simulink model "AlexFullVehicleModel2018"  (R2018b)
settings: Solver=FixedStepAuto  StartTime=0.0  StopTime=20  FixedStep=global_time_step  MaxStep=0.05  RelTol=1e-3
values from neighbouring files (symbols this model uses):
  B_lat = @(i,u,v)feval(B_surf_lat{i},[u,v])    [initfunctions.m]
  B_long = @(i,u,v)feval(B_surf_long{i},[u,v])    [initfunctions.m]
  brake_bias = 0.6    [fvm_parameters.m]
  brake_pad_radius = 0.1    [fvm_parameters.m]
  C_lat = @(i,u,v)feval(C_surf_lat{i},[u,v])    [initfunctions.m]
  C_long = @(i,u,v)feval(C_surf_long{i},[u,v])    [initfunctions.m]
  D_lat = @(i,u,v)feval(D_surf_lat{i},[u,v])    [initfunctions.m]
  D_long = @(i,u,v)feval(D_surf_long{i},[u,v])    [initfunctions.m]
  E_lat = @(i,u,v)feval(E_surf_lat{i},[u,v])    [initfunctions.m]
  E_long = @(i,u,v)feval(E_surf_long{i},[u,v])    [initfunctions.m]
  front_piston_area = 1.555284713E-3    (= 0.001555284713)    [fvm_parameters.m]
  master_cylinder_area = 3.3329E-4    (= 0.00033329)    [fvm_parameters.m]
  mu_brake = 0.35    [fvm_parameters.m]
  Mu_lat = @(i,u,v)feval(Mu_surf_lat{i},[u,v])    [initfunctions.m]
  Mu_long = @(i,u,v)feval(Mu_surf_long{i},[u,v])    [initfunctions.m]
  n_pads = 2    [fvm_parameters.m]
  pedal_ratio = 5.22    [fvm_parameters.m]
  rear_piston_area = 1.017876020E-3    (= 0.00101787602)    [fvm_parameters.m]
undefined symbols (not defined in the file or in its folder): sigbuilder_block
libraries: cstblocks x1
settings Model: Creator=jbray  LastModifiedBy=univ4123
settings SolverCC: InitialStep=0.001
settings DataIOCC: ReturnWorkspaceOutputs=on
settings DebuggingCC: UnderSpecifiedDimensionMsg=warning

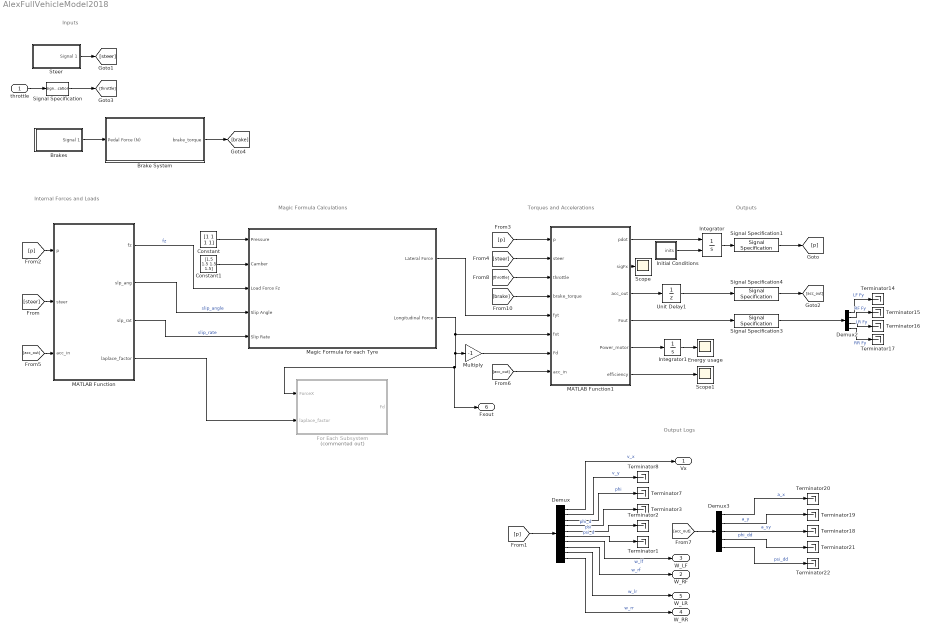
== system AlexFullVehicleModel2018 ==
  note: Torques and Accelerations
  note: Internal Forces and Loads
  note: Outputs
  note: Output Logs
  note: Magic Formula Calculations
  note: Inputs
  throttle : Inport
  Brake System : Subsystem
  Brakes : Subsystem  Tag=STV Subsys  LoadFcn=sigbuilder_block('load');  StartFcn=sigbuilder_block('start');  StopFcn=sigbuilder_block('stop');  ClipboardFcn=sigbuilder_block('clipboard');  mask(Sigbuilder block){tuvar=[0:10]}
      mask help: Simulink:masks:SigbuilderBlock_MD
      mask init:
      | if ~strcmp(get_param(bdroot(gcbh),'SimulationStatus'),'stopped') tuvar = sigbuilder_block('maskInit'); end
      settings: CopyFcn=sigbuilder_block('copy');  DeleteFcn=sigbuilder_block('delete');  ModelCloseFcn=sigbuilder_block('modelClose');  PreSaveFcn=sigbuilder_block('preSave');  PauseFcn=sigbuilder_block('pause');  ContinueFcn=sigbuilder_block('continue');  NameChangeFcn=sigbuilder_block('namechange');  OpenFcn=sigbuilder_block('open',[404 117.5 550.5 362.5 ]);  CloseFcn=sigbuilder_block('close');
      mask Display: plot(0, 0, 100, 100,[2, 2, 32, 32, 2], [68, 8, 8, 68, 68],[32, 2], [38, 38], [32, 19, 2],[53, 60, 44], [32, 17, 17, 2],[16, 16, 31, 31]);txt = getActiveGroup(gcbh);text(2, 100, txt,'verticalAlignment', 'top');
  Constant : Constant  Value=[1 1 1 1]  VectorParams1D=off  LockScale=on
  Constant1 : Constant  Value=[1.5 1.5 1.5 1.5]  VectorParams1D=off  LockScale=on
  Demux : Demux  Outputs=10
  Demux2 : Demux
  Demux3 : Demux  Outputs=5
  Energy usage : Scope
  For Each Subsystem : Subsystem  Commented=on  TreatAsAtomicUnit=on
  "Initial Conditions " : Subsystem
  Integrator : Integrator  InitialConditionSource=external
  Integrator1 : Integrator
  MATLAB Function : MATLAB Function  TreatAsAtomicUnit=on
  MATLAB Function1 : MATLAB Function  TreatAsAtomicUnit=on
  Magic Formula for each Tyre : Subsystem  TreatAsAtomicUnit=on
  Multiply : Gain  Gain=-1
  Scope : Scope
  Scope1 : Scope
  Signal Specification : SignalSpecification  Dimensions=[2,1]
  Signal Specification1 : SignalSpecification  Dimensions=10
  Signal Specification3 : SignalSpecification  Dimensions=4
  Signal Specification4 : SignalSpecification  Dimensions=5
  "Steer " : Subsystem  Tag=STV Subsys  LoadFcn=sigbuilder_block('load');  StartFcn=sigbuilder_block('start');  StopFcn=sigbuilder_block('stop');  ClipboardFcn=sigbuilder_block('clipboard');  mask(Sigbuilder block){tuvar=[0:10]}
      mask help: Simulink:masks:SigbuilderBlock_MD
      mask init:
      | if ~strcmp(get_param(bdroot(gcbh),'SimulationStatus'),'stopped') tuvar = sigbuilder_block('maskInit'); end
      settings: CopyFcn=sigbuilder_block('copy');  DeleteFcn=sigbuilder_block('delete');  ModelCloseFcn=sigbuilder_block('modelClose');  PreSaveFcn=sigbuilder_block('preSave');  PauseFcn=sigbuilder_block('pause');  ContinueFcn=sigbuilder_block('continue');  NameChangeFcn=sigbuilder_block('namechange');  OpenFcn=sigbuilder_block('open',[404 117.5 550.5 362.5 ]);  CloseFcn=sigbuilder_block('close');
      mask Display: plot(0, 0, 100, 100,[2, 2, 32, 32, 2], [68, 8, 8, 68, 68],[32, 2], [38, 38], [32, 19, 2],[53, 60, 44], [32, 17, 17, 2],[16, 16, 31, 31]);txt = getActiveGroup(gcbh);text(2, 100, txt,'verticalAlignment', 'top');
  Terminator{1..3,7..8,14..22} (14 alike) : Terminator
  Unit Delay1 : UnitDelay  SampleTime=-1
  Vx : Outport
  W_RF : Outport  Port=2
  W_LF : Outport  Port=3
  W_RR : Outport  Port=4
  W_LR : Outport  Port=5
  Fxout : Outport  Port=6
  wires:
  MATLAB Function1/1(pdot) -> Integrator/1
  Integrator/1 -> Signal Specification1/1
  Demux/10 -> W_RR/1  "w_rr"
  Demux/9 -> W_LR/1  "w_lr"
  Demux/6 -> Terminator1/1  "psi_d"
  Demux/5 -> Terminator2/1  "psi"
  Demux/4 -> Terminator3/1  "phi_d"
  Demux/7 -> W_LF/1  "w_lf"
  Demux/8 -> W_RF/1  "w_rf"
  Demux/3 -> Terminator7/1  "phi"
  Demux/2 -> Terminator8/1  "v_y"
  Demux/1 -> Vx/1  "v_x"
  Demux2/4 -> Terminator17/1  "RR Fy"
  Demux2/3 -> Terminator16/1  "LR Fy"
  Demux2/2 -> Terminator15/1  "RF Fy"
  Demux2/1 -> Terminator14/1  "LF Fy"
  Signal Specification3/1 -> Demux2/1
  Demux3/3 -> Terminator18/1  "a_sy"
  Demux3/2 -> Terminator19/1  "a_y"
  Demux3/1 -> Terminator20/1  "a_x"
  Demux3/4 -> Terminator21/1  "phi_dd"
  Demux3/5 -> Terminator22/1  "psi_dd"
  MATLAB Function/3(slp_rat) -> Magic Formula for each Tyre/5(Slip Rate)  "slip_rate"
  MATLAB Function/1(fz) -> Magic Formula for each Tyre/3(Load Force Fz)  "fz"
  Constant/1 -> Magic Formula for each Tyre/1(Pressure)
  Magic Formula for each Tyre/1(Lateral Force) -> MATLAB Function1/5(fyt)
  Magic Formula for each Tyre/2(Longitudinal Force) -> MATLAB Function1/6(fxt), Multiply/1, Fxout/1, For Each Subsystem/1(ForceX)
  MATLAB Function1/3(acc_out) -> Unit Delay1/1
  MATLAB Function/2(slp_ang) -> Magic Formula for each Tyre/4(Slip Angle)  "slip_angle"
  Constant1/1 -> Magic Formula for each Tyre/2(Camber)
  MATLAB Function1/2(sigFx) -> Scope/1
  MATLAB Function/4(laplace_factor) -> For Each Subsystem/2(laplace_factor)
  Signal Specification1/1 -> [p]
  [p] -> Demux/1
  [p] -> MATLAB Function/1(p)
  [p] -> MATLAB Function1/1(p)
  [steer] -> MATLAB Function/2(steer)
  [steer] -> MATLAB Function1/2(steer)
  Unit Delay1/1 -> Signal Specification4/1
  Signal Specification4/1 -> [acc_out]
  [acc_out] -> MATLAB Function/3(acc_in)
  [acc_out] -> MATLAB Function1/8(acc_in)
  [acc_out] -> Demux3/1
  "Initial Conditions "/1("inits ") -> Integrator/2
  Multiply/1 -> MATLAB Function1/7(Fd)
  [throttle] -> MATLAB Function1/3(throttle)
  MATLAB Function1/5(Power_motor) -> Integrator1/1
  Integrator1/1 -> Energy usage/1
  MATLAB Function1/6(efficiency) -> Scope1/1
  "Steer "/1(Signal 1) -> [steer]
  throttle/1 -> Signal Specification/1
  Brakes/1(Signal 1) -> Brake System/1(Pedal Force (N))
  Brake System/1("brake_torque ") -> [brake]
  [brake] -> MATLAB Function1/4(brake_torque)
  MATLAB Function1/4(Fout) -> Signal Specification3/1
  Signal Specification/1 -> [throttle]

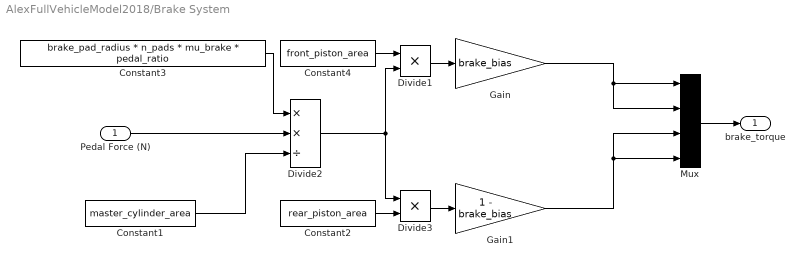
== system AlexFullVehicleModel2018/Brake System ==
  Pedal Force (N) : Inport
  Constant1 : Constant  Value=master_cylinder_area
  Constant2 : Constant  Value=rear_piston_area
  Constant3 : Constant  Value=brake_pad_radius * n_pads * mu_brake * pedal_ratio
  Constant4 : Constant  Value=front_piston_area
  Divide1 : Product
  Divide2 : Product  Inputs=**/
  Divide3 : Product
  Gain : Gain  Gain=brake_bias
  Gain1 : Gain  Gain=1 - brake_bias
  Mux : Mux
  "brake_torque " : Outport
  wires:
  Mux/1 -> "brake_torque "/1
  Divide1/1 -> Gain/1
  Pedal Force (N)/1 -> Divide2/2
  Constant1/1 -> Divide2/3
  Constant2/1 -> Divide3/2
  Divide2/1 -> Divide1/2, Divide3/1
  Divide3/1 -> Gain1/1
  Constant3/1 -> Divide2/1
  Gain/1 -> Mux/2, Mux/1
  Constant4/1 -> Divide1/1
  Gain1/1 -> Mux/4, Mux/3

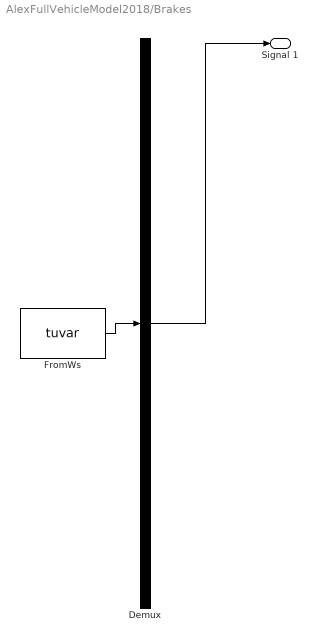
== system AlexFullVehicleModel2018/Brakes ==
  Demux : Demux  Tag=STV Demux  Outputs=1
  FromWs : FromWorkspace  Tag=STV FromWs  VariableName=tuvar  SampleTime=0
      SigBuilderData=|
      | common.afterFinalStr = 'Extrapolate'
      | common.sampleTime = 0
      | dataSet.timeRange = [0 20]
      | dataSet.name = 'Group 1'
      | sbobj.Groups.Name = 'Group 1'
      | sbobj.Groups.Signals.Name = 'Signal 1'
      | sbobj.Groups.Signals.XData = [0 9.02 14 17.25 20]
      | sbobj.Groups.Signals.YData = [0 0 0 0 0]
      | sbobj.Groups.TimeRange = [0 20]
  Signal 1 : Outport  Tag=STV Outport
  wires:
  Demux/1 -> Signal 1/1
  FromWs/1 -> Demux/1

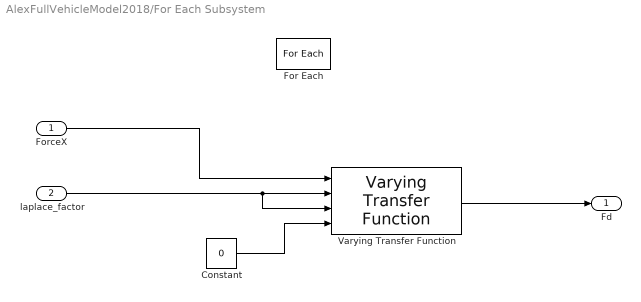
== system AlexFullVehicleModel2018/For Each Subsystem ==
  ForceX : Inport  Partition=on  PartitionDimension=1  PartitionWidth=1  PartitionOffset=0
  laplace_factor : Inport  Port=2  Partition=on  PartitionDimension=2  PartitionWidth=1  PartitionOffset=0
  Constant : Constant  Value=0
  For Each : ForEach  DisableCoverage=on  IndexMode=One-based
  Varying Transfer Function : cstblocks/Linear Parameter Varying/Varying Transfer Function  N=1
      settings: SourceProductName=Control System Toolbox
  "Fd " : Outport  ConcatenationDimension=1
  wires:
  Constant/1 -> Varying Transfer Function/4
  laplace_factor/1 -> Varying Transfer Function/3, Varying Transfer Function/2
  ForceX/1 -> Varying Transfer Function/1
  Varying Transfer Function/1 -> "Fd "/1

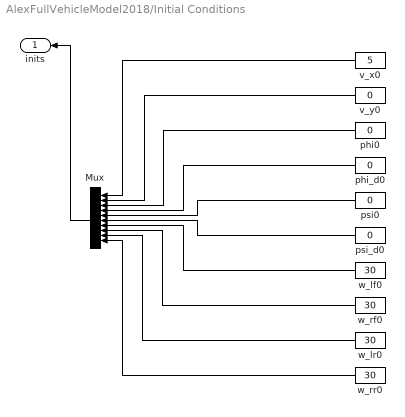
== system AlexFullVehicleModel2018/Initial Conditions  ==
  Mux : Mux  Inputs=10
  phi0 : Constant  Value=0
  phi_d0 : Constant  Value=0
  psi0 : Constant  Value=0
  psi_d0 : Constant  Value=0
  v_x0 : Constant  Value=5
  v_y0 : Constant  Value=0
  w_lf0 : Constant  Value=30
  w_lr0 : Constant  Value=30
  w_rf0 : Constant  Value=30
  w_rr0 : Constant  Value=30
  "inits " : Outport
  wires:
  w_lf0/1 -> Mux/7
  Mux/1 -> "inits "/1
  psi_d0/1 -> Mux/6
  psi0/1 -> Mux/5
  phi_d0/1 -> Mux/4
  phi0/1 -> Mux/3
  v_y0/1 -> Mux/2
  w_rf0/1 -> Mux/8
  v_x0/1 -> Mux/1
  w_rr0/1 -> Mux/10
  w_lr0/1 -> Mux/9

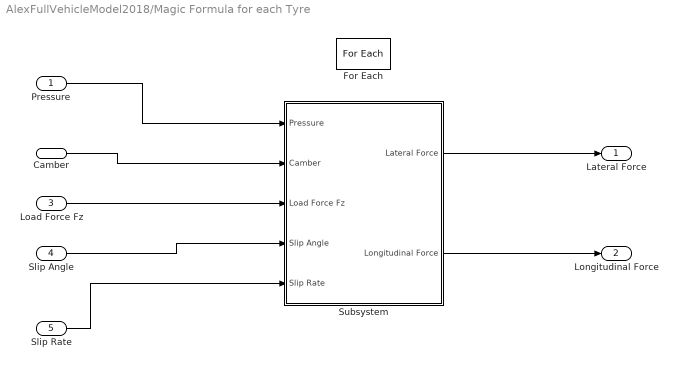
== system AlexFullVehicleModel2018/Magic Formula for each Tyre ==
  Pressure : Inport  Partition=on  PartitionDimension=2  PartitionWidth=1  PartitionOffset=0
  Camber : Inport  Port=2  Partition=on  PartitionDimension=2  PartitionWidth=1  PartitionOffset=0
  Load Force Fz : Inport  Port=3  Partition=on  PartitionDimension=2  PartitionWidth=1  PartitionOffset=0
  Slip Angle : Inport  Port=4  Partition=on  PartitionDimension=2  PartitionWidth=1  PartitionOffset=0
  Slip Rate : Inport  Port=5  Partition=on  PartitionDimension=2  PartitionWidth=1  PartitionOffset=0
  For Each : ForEach  DisableCoverage=on  IndexMode=One-based
  Subsystem : Subsystem
  Lateral Force : Outport  ConcatenationDimension=1
  Longitudinal Force : Outport  Port=2  ConcatenationDimension=1
  wires:
  Slip Rate/1 -> Subsystem/5(Slip Rate)
  Slip Angle/1 -> Subsystem/4(Slip Angle)
  Pressure/1 -> Subsystem/1(Pressure)
  Subsystem/1(Lateral Force) -> Lateral Force/1
  Load Force Fz/1 -> Subsystem/3(Load Force Fz)
  Camber/1 -> Subsystem/2(Camber)
  Subsystem/2(Longitudinal Force) -> Longitudinal Force/1

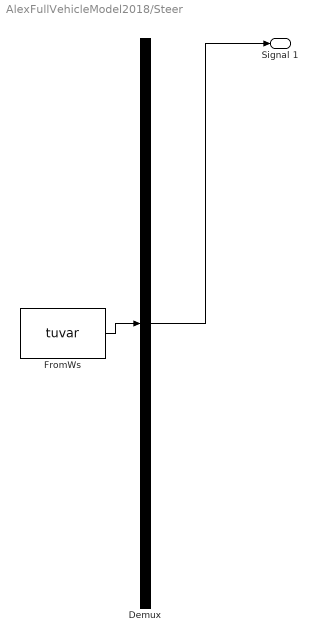
== system AlexFullVehicleModel2018/Steer  ==
  Demux : Demux  Tag=STV Demux  Outputs=1
  FromWs : FromWorkspace  Tag=STV FromWs  VariableName=tuvar  SampleTime=0
      SigBuilderData=|
      | common.afterFinalStr = 'Extrapolate'
      | common.sampleTime = 0
      | dataSet.timeRange = [0 20]
      | dataSet.name = 'Group 1'
      | sbobj.Groups.Name = 'Group 1'
      | sbobj.Groups.Signals.Name = 'Signal 1'
      | sbobj.Groups.Signals.XData = [0 4 6 16 20]
      | sbobj.Groups.Signals.YData = [0 0 0 0 0]
      | sbobj.Groups.TimeRange = [0 20]
  Signal 1 : Outport  Tag=STV Outport
  wires:
  Demux/1 -> Signal 1/1
  FromWs/1 -> Demux/1

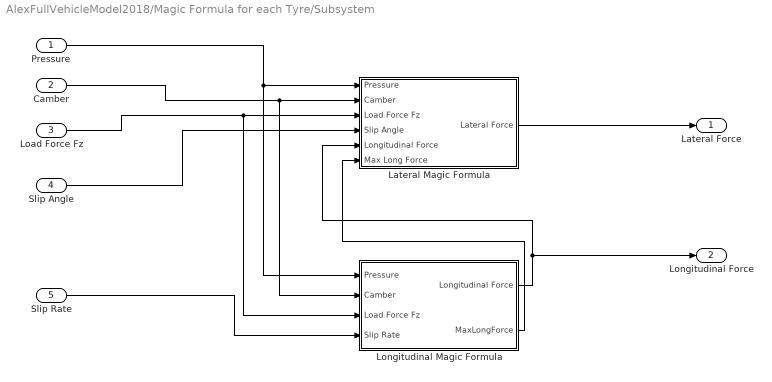
== system AlexFullVehicleModel2018/Magic Formula for each Tyre/Subsystem ==
  Pressure : Inport
  Camber : Inport  Port=2
  Load Force Fz : Inport  Port=3
  Slip Angle : Inport  Port=4
  Slip Rate : Inport  Port=5
  Lateral Magic Formula : Subsystem
  Longitudinal Magic Formula : Subsystem
  Lateral Force : Outport
  Longitudinal Force : Outport  Port=2
  wires:
  Slip Angle/1 -> Lateral Magic Formula/4(Slip Angle)
  Lateral Magic Formula/1(Lateral Force) -> Lateral Force/1
  Load Force Fz/1 -> Longitudinal Magic Formula/3(Load Force Fz), Lateral Magic Formula/3(Load Force Fz)
  Longitudinal Magic Formula/1(Longitudinal Force) -> Lateral Magic Formula/5(Longitudinal Force), Longitudinal Force/1
  Camber/1 -> Longitudinal Magic Formula/2(Camber), Lateral Magic Formula/2(Camber)
  Slip Rate/1 -> Longitudinal Magic Formula/4(Slip Rate)
  Pressure/1 -> Longitudinal Magic Formula/1(Pressure), Lateral Magic Formula/1(Pressure)
  Longitudinal Magic Formula/2("MaxLongForce ") -> Lateral Magic Formula/6(Max Long Force)

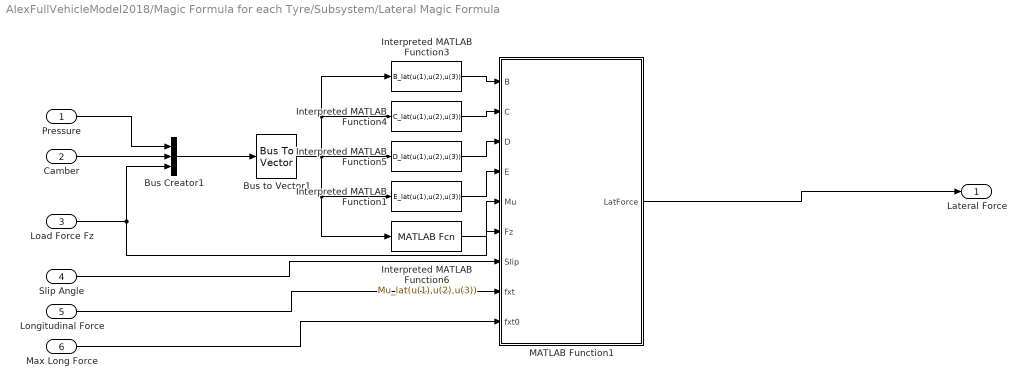
== system AlexFullVehicleModel2018/Magic Formula for each Tyre/Subsystem/Lateral Magic Formula ==
  Pressure : Inport
  Camber : Inport  Port=2
  Load Force Fz : Inport  Port=3
  Slip Angle : Inport  Port=4
  Longitudinal Force : Inport  Port=5
  Max Long Force : Inport  Port=6
  Bus Creator1 : BusCreator  Inputs=3
  Bus to Vector1 : BusToVector
  Interpreted MATLAB Function1 : MATLABFcn  MATLABFcn=E_lat(u(1),u(2),u(3))
  Interpreted MATLAB Function3 : MATLABFcn  MATLABFcn=B_lat(u(1),u(2),u(3))
  Interpreted MATLAB Function4 : MATLABFcn  MATLABFcn=C_lat(u(1),u(2),u(3))
  Interpreted MATLAB Function5 : MATLABFcn  MATLABFcn=D_lat(u(1),u(2),u(3))
  Interpreted MATLAB Function6 : MATLABFcn  MATLABFcn=Mu_lat(u(1),u(2),u(3))
  MATLAB Function1 : MATLAB Function  TreatAsAtomicUnit=on
  Lateral Force : Outport
  wires:
  Interpreted MATLAB Function3/1 -> MATLAB Function1/1(B)
  Interpreted MATLAB Function1/1 -> MATLAB Function1/4(E)
  Bus to Vector1/1 -> Interpreted MATLAB Function1/1, Interpreted MATLAB Function6/1, Interpreted MATLAB Function3/1, Interpreted MATLAB Function4/1, Interpreted MATLAB Function5/1
  Load Force Fz/1 -> Bus Creator1/3, MATLAB Function1/6(Fz)
  Interpreted MATLAB Function4/1 -> MATLAB Function1/2(C)
  Slip Angle/1 -> MATLAB Function1/7(Slip)
  Interpreted MATLAB Function5/1 -> MATLAB Function1/3(D)
  Pressure/1 -> Bus Creator1/1
  Interpreted MATLAB Function6/1 -> MATLAB Function1/5(Mu)
  Bus Creator1/1 -> Bus to Vector1/1
  Camber/1 -> Bus Creator1/2
  MATLAB Function1/1(LatForce) -> Lateral Force/1
  Longitudinal Force/1 -> MATLAB Function1/8(fxt)
  Max Long Force/1 -> MATLAB Function1/9(fxt0)

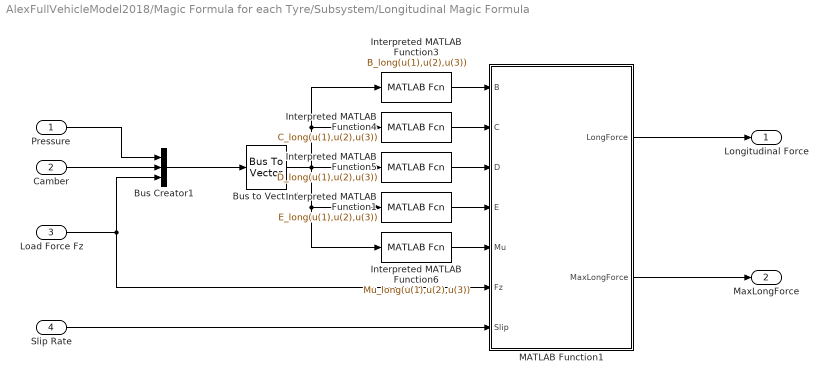
== system AlexFullVehicleModel2018/Magic Formula for each Tyre/Subsystem/Longitudinal Magic Formula ==
  Pressure : Inport
  Camber : Inport  Port=2
  Load Force Fz : Inport  Port=3
  Slip Rate : Inport  Port=4
  Bus Creator1 : BusCreator  Inputs=3
  Bus to Vector1 : BusToVector
  Interpreted MATLAB Function1 : MATLABFcn  MATLABFcn=E_long(u(1),u(2),u(3))
  Interpreted MATLAB Function3 : MATLABFcn  MATLABFcn=B_long(u(1),u(2),u(3))
  Interpreted MATLAB Function4 : MATLABFcn  MATLABFcn=C_long(u(1),u(2),u(3))
  Interpreted MATLAB Function5 : MATLABFcn  MATLABFcn=D_long(u(1),u(2),u(3))
  Interpreted MATLAB Function6 : MATLABFcn  MATLABFcn=Mu_long(u(1),u(2),u(3))
  MATLAB Function1 : MATLAB Function  TreatAsAtomicUnit=on
  Longitudinal Force : Outport
  "MaxLongForce " : Outport  Port=2
  wires:
  Interpreted MATLAB Function3/1 -> MATLAB Function1/1(B)
  Interpreted MATLAB Function1/1 -> MATLAB Function1/4(E)
  Bus to Vector1/1 -> Interpreted MATLAB Function1/1, Interpreted MATLAB Function6/1, Interpreted MATLAB Function3/1, Interpreted MATLAB Function4/1, Interpreted MATLAB Function5/1
  Load Force Fz/1 -> Bus Creator1/3, MATLAB Function1/6(Fz)
  MATLAB Function1/1(LongForce) -> Longitudinal Force/1
  Interpreted MATLAB Function4/1 -> MATLAB Function1/2(C)
  Slip Rate/1 -> MATLAB Function1/7(Slip)
  Interpreted MATLAB Function5/1 -> MATLAB Function1/3(D)
  Pressure/1 -> Bus Creator1/1
  Interpreted MATLAB Function6/1 -> MATLAB Function1/5(Mu)
  Bus Creator1/1 -> Bus to Vector1/1
  Camber/1 -> Bus Creator1/2
  MATLAB Function1/2(MaxLongForce) -> "MaxLongForce "/1

== matlab function AlexFullVehicleModel2018/MATLAB Function1 ==
  data: p input; pdot output; sigFx output; steer input; throttle input; brake_torque input; fyt input size=4; fxt input size=4; Fd input; acc_in input; acc_out output size=5; Fout output; Power_motor output; efficiency output; param parameter
function [pdot,sigFx,acc_out,Fout,Power_motor,efficiency] = fcn(p,steer,throttle,brake_torque,fyt,fxt,Fd,acc_in,param)

%% Output
pdot=zeros(10,1);

%% Constant
g = 9.81; %acceleration due to gravity
    
%% Functions


%% Current States
v_x = p(1); %x velocity (m/s)
v_y = p(2); %y velocity (m/s)
phi = p(3); %phi (roll) (rad)
phi_d = p(4); %d(phi)/dt (roll rate) (rad/s)
psi = p(5); %psi (yaw) (rad)
psi_d = p(6); %d(psi)/dt (yaw rate) (rad/s)
a_x = acc_in(1); %x acceleration (m/s^2)
a_y = acc_in(2); %y accelerarion (m/s^2)
phi_dd = acc_in(4); %d^2(phi)/dt^2 (rad/s^2)
psi_dd = acc_in(5); %d^2(psi)/dt^2 (rad/s^2)

om = zeros([1,4]);

for i = 7:10

    om(i-6) = p(i); %angular speed of wheels (rad/s)

end
%% Car Physical Variables

l_fs = param.l_fs; %distance from front axle to sprung centre of mass (m)
l_rs = param.l_rs; %distance from rear axle to sprung centre of mass (m)
t_f = param.t_f; %front wheel track (m)
t_r = param.t_r; %rear wheel track (m)
h_f = param.h_f; %height of roll axis above ground at front axle (m)
h_r = param.h_r; %height of roll axis above ground at rear axle (m)
h_cgs = param.h_cgs; %height of sprung centre of mass above ground (m)
h_cguf = param.h_cguf; %height of front unsprung centre of mass above ground (m)
h_cgur = param.h_cgur; %height of rear unsprung centre of mass above ground (m)
M = param.M; %total mass (sprung + unsprung) (kg)
M_uf = param.M_uf; %front unsprung mass (kg) (I think of this is combined left and right)
M_ur = param.M_ur; %rear unsprung mass (kg)
I_xxs = param.I_xxs;    %
I_xys = param.I_xys;          %
I_xzs = param.I_xzs;    %sprung mass moment
I_yys = param.I_yys;   %of inertia tensor
I_yzs = param.I_yzs;          %
I_zzs = param.I_zzs;    %
I_zzuf = param.I_zzuf; %front unsprung mass moment of inertia
I_zzur = param.I_zzur; %rear unsprung mass moment of inertia
I_tlf = param.I_tlf; %
I_trf = param.I_trf; %moment of inertia of tyres
I_tlr = param.I_tlr; %(and I guess wheels too)
I_trr = param.I_trr; %

%spring/dampers
K_spf = param.K_spf; %front suspension stiffness (N/mm)
K_spr = param.K_spr; %rear suspension stiffness (N/mm)
B_f = param.B_f; %front suspension damping (Ns/mm)
B_r = param.B_r; %rear suspension damping (Ns/mm)

%anti-roll bars
K_rf = param.K_rf; %front anti-roll bar stiffness (Nm/rad)
K_rr = param.K_rr; %rear anti-roll bar stiffness (Nm/rad)

%roll stiffness
K_phif = param.K_phif; %(Nm/rad) not sure what 0.766 and 0.827 are
K_phir = param.K_phir; %(Nm/rad)
K_phi = param.K_phi;

%roll damping
B_phif = param.B_phif; %(Nms/rad) again, not sure about 0.766 and 0.827
B_phir = param.B_phir; %(Nms/rad)

K_sr = param.K_sr; %steering-to-wheel angle ratio (1/deg)

%tyre properties
t_wid = param.t_wid; %tyre width (m)
t_rad = param.t_rad; %tyre outer radius (m)
t_pressure = param.t_pressure; %tyre pressure (Pa)

Ax = param.Ax;% surface area for drag
Ay = param.Ay;

rho = param.rho; %air density
c_drag = param.c_drag; %drag coefficient

%% Calculated Parameters
L = l_fs + l_rs; %wheelbase (m)
M_s = M - M_uf - M_ur; %sprung mass (kg) maybe should be factor of 2 in there???
l_cgs = (M_ur*l_rs - M_uf*l_fs)/M; %distance from total centre of mass to sprung centre of mass (m)
l_f = l_fs + l_cgs; %distance between front axle and total centre of mass (m)
l_r = l_rs - l_cgs; %distance between rear axle and total centre of mass (m)
M_f = M*l_r/L; %mass on front axle (kg)
M_r = M*l_f/L; %mass on reat axle (kg)
h_o = h_f + l_f*(h_r - h_f)/L; %height of roll axis above ground at total centre of mass (m)
h_s = h_cgs - h_o; %height of sprung centre of mass above roll axis (m)
h_uf = h_cguf - h_o; %height of front unsprung centre of mass above roll axis (m)
h_ur = h_cgur - h_o; %height of rear unsprung centre of mass above roll axis (m)
h_cg = (M_s*h_cgs + M_uf*h_cguf + M_ur*h_cgur)/M; %height of total centre of mass above ground (m)

%% Steering Inputs
d_steer = steer; %gets steering input

%% Calculate Internal Accelerations
%(V_0y = 0)

a_sy = psi_d*v_x + l_cgs*psi_dd + h_s*cos(phi)*phi_dd - h_s*phi_d^2*sin(phi) - h_s*psi_d^2*sin(phi); %sprung mass y-acceleration (eqn 2.29)

%%a_ufx = a_x - l_f*psi_d^2; %front unsprung mass x-acceleration (eqn 2.16)
%%a_ufy = a_y + l_f*psi_dd; %front unsprung mass y-acceleration (eqn 2.16)
%%a_urx = a_x + l_r*psi_d^2; %rear unsprung mass x-acceleration (eqn 2.22)
%%a_ury = a_y - l_r*psi_dd; %rear unsprung mass y-acceleration (eqn 2.22)

%% Rotation Matrix
ROT = [1,0,0;...
    0,cos(phi),sin(phi);...
    0,-sin(phi),cos(phi)]; %eqn 2.39
I_b = [I_xxs+M_s*h_s^2,I_xys,I_xzs+M_s*h_s*l_cgs;...
    I_xys,I_yys+M_s*(h_s^2+l_cgs^2),I_yzs;...
    I_xzs+M_s*h_s*l_cgs,I_yzs,I_zzs+M_s*l_cgs^2]; %sprung mass inertia tensor (eqn 2.38)

I_c = ROT*I_b*ROT'; %chassis inertia tensor (eqn 2.40)
I_zzus = M_uf*l_f^2 + M_ur*l_r^2 + I_zzuf + I_zzur; %eqn 2.41
I_xxo = I_c(1,1);
I_zzo = I_c(3,3) + I_zzus; %effective I_zz (eqn 2.42)

%% Dynamic Weight Transfer Forces

%% Tyre Longitudinal/Lateral Forces
%left front wheel velocity  %
v_xlf = v_x + psi_d*t_f/2;  %
v_ylf = v_y + psi_d*l_f;    %
                            %
%right front wheel velocity %
v_xrf = v_x - psi_d*t_f/2;  %
v_yrf = v_y + psi_d*l_f;    %look at rotation (yaw) of car and draw triangles
                            %to see where these expressions come from
%left rear wheel velocity   %
v_xlr = v_x + psi_d*t_r/2;  %
v_ylr = v_y - psi_d*l_r;    %
                            %
%right rear wheel velocity  %
v_xrr = v_x - psi_d*t_r/2;  %
v_yrr = v_y - psi_d*l_r;    %

v_xA = [v_xlf,v_xrf,v_xlr,v_xrr]; 
v_yA = [v_ylf,v_yrf,v_ylr,v_yrr];


%tyre updates
% omega_lf = (v_xlf^2 + v_ylf^2)^(1/2); %
% omega_rf = (v_xrf^2 + v_yrf^2)^(1/2); %new wheel speeds
% omega_lr = (v_xlr^2 + v_ylr^2)^(1/2); %(omega is a misleading name)
% omega_rr = (v_xrr^2 + v_yrr^2)^(1/2); %

%get steering angle
delta = d_steer*pi/(180*K_sr); %gets steering angle from input (rad)

Fxlf = fxt(1)*cos(delta) - fyt(1)*sin(delta); %
Fxrf = fxt(2)*cos(delta) - fyt(2)*sin(delta); %
Fxlr = fxt(3);                               %
Fxrr = fxt(4);                               %converts tyre frame forces into
Fylf = fyt(1)*cos(delta) + fxt(1)*sin(delta); %(non-rotating) body frame
Fyrf = fyt(2)*cos(delta) + fxt(2)*sin(delta); %
Fylr = fyt(3);                               %
Fyrr = fyt(4);                               %
Fout1 = [Fylf,Fyrf,Fylr,Fyrr]; %outputs tyre forces
Fout = Fout1(:);
%Fout.x = [Fxlf,Fxrf,Fxlr,Fxrr];
Mzlf = 0; %
Mzrf = 0; %self-aligning torque of wheels (Nm)
Mzlr = 0; %
Mzrr = 0; %

%Omeaga/Alpha of Wheels
torque_total=zeros([1,4]);
Td = zeros([1 4]);
motor_torque = zeros([1,4]);

r_coeffs = [157.6658 -0.2740];%these are speed vs. torque linear regression coeffs b0, b1
b0 = r_coeffs(1);
b1 = r_coeffs(2);
gear_ratio = 5;

if om(3)*5 < 575
    motor_torque(3) = gear_ratio*throttle(1)*(b0+b1*om(3)*gear_ratio); %apply regression
else
    motor_torque(3) = 0; %ensures no negative motor torques
end

if om(4)*5 < 575
    motor_torque(4) = gear_ratio*throttle(2)*(b0+b1*om(4)*gear_ratio); %apply regression
else
    motor_torque(4) = 0;
end

My = zeros([1,4]); %self-aligning torque, to be added to the model later
Power_motor = zeros([1,4]);
efficiency = zeros([1,4]);

roll_resist_coeff = 0.0001;


%%efficiency coeffs
%%from a 2 exponential fit of the efficiency curve of the motor

a =  -3.163e-14;
b =     0.00639;
c =       42.49;
d =   0.0001557;

rpm_conversion = 9.5493;

%%torque and motor

for i = 1:4
    
    Td(i) = Fd(i)*t_rad; %%torque against rotation due to longitudinal force from tyres
    
    torque_total(i) = motor_torque(i) + Td(i) - brake_torque(i) - roll_resist_coeff*om(i); %Td is the road-tyre response torque
    
    efficiency(i) = a*exp(b*5*om(i)*rpm_conversion) + c*exp(d*5*om(i)*rpm_conversion); %applying the exponential fit
    Power_motor(i) =  (abs(om(i))*abs(motor_torque(i)))/(efficiency(i)*0.01); %calculating the power requirement
end

alpha_lf_new = torque_total(1)/I_tlf; %
alpha_rf_new = torque_total(2)/I_trf; %angular acceleration of wheels (rad/s^2)
alpha_lr_new = torque_total(3)/I_tlr; %
alpha_rr_new = torque_total(4)/I_trr; %

%% Torques
T_phif = -K_phif*phi - B_phif*phi_d; %front rolling torque (eqn 2.48)
T_phir = -K_phir*phi - B_phir*phi_d; %rear rolling torque (eqn 2.48)

%% Sum forces and torques
sigFx = Fxlf + Fxrf + Fxlr + Fxrr -  (sign(v_x)*((1/2)*c_drag*rho*Ax*(v_x^2))); %total x-force (eqn 2.35) add drag here???
sigFy = Fylf + Fyrf + Fylr + Fyrr; %total y-force (eqn 2.36)
sigTxs = T_phif + T_phir - M_s*g*h_s*sin(phi) + M_s*h_s*a_sy*cos(phi); %total torque about x-axis (roll) (eqn 2.47)
sigTz = (Fylf + Fyrf)*l_f - (Fylr + Fyrr)*l_r + t_f/2*(Fxlf - Fxrf) + t_r/2*(Fxlr - Fxrr) + Mzlf + Mzrf + Mzlr + Mzrr; %total torque about z-axis (yaw) (eqn 2.49)
    
%% Update Independent Variables
a_x_new = (sigFx + M_s.*(-2*h_s.*phi_d.*psi_d.*cos(phi) - h_s.*psi_dd.*sin(phi)))./M; %new x-acceleration (eqn 2.33)
a_y_new = (sigFy - M_s*(-h_s*phi_dd*cos(phi) + h_s*phi_d^2*sin(phi) + h_s*psi_d^2*sin(phi)))./M; %new y-acceleration (eqn 2.34)
phi_dd_new = (sigTxs - (I_xzs+M_s*h_s*l_cgs)*cos(phi)*psi_dd + (I_xzs+M_s*h_s*l_cgs)*sin(phi)*phi_d*psi_d + (I_zzs - I_yys - M_s*h_s^2)*sin(phi)*cos(phi)*psi_d^2)./(I_xxs+M_s*h_s^2); %new d^2(phi)/dt^2 (eqn 2.45)
psi_dd_new = (sigTz - (I_xzs+M_s*h_s*l_cgs)*cos(phi)*phi_dd - (I_xzs+M_s*h_s*l_cgs)*sin(phi)*phi_d^2 - M_s*h_s*a_x*sin(phi) - (I_zzs - I_yys - M_s*h_s^2)*sin(phi)*cos(phi)*psi_d*phi_d)./I_zzo; %new d^2(psi)/dt^2 (eqn 2.46)

%acceleration outputs
acc_out_1 = [a_x_new,a_y_new,a_sy,phi_dd_new,psi_dd_new]; %outputs new acceleraltions
acc_out = acc_out_1(:);
%% Outputs (derivative of) new state information
%X
pdot(1) = a_x_new;

%Y
pdot(2) = a_y_new;

%PHI
pdot(3) = phi_d;
pdot(4) = phi_dd_new;

%PSI
pdot(5) = psi_d;
pdot(6) = psi_dd_new;

%WHEELS
pdot(7) = alpha_lf_new;
pdot(8) = alpha_rf_new;
pdot(9) = alpha_lr_new;
pdot(10) = alpha_rr_new;

== matlab function AlexFullVehicleModel2018/MATLAB Function ==
  data: fz output; p input; steer input; acc_in input; slp_ang output; slp_rat output; laplace_factor output; param parameter
function [fz,slp_ang,slp_rat,laplace_factor] = fcn(p,steer,acc_in,param)


%% Constant
g = 9.81; %acceleration due to gravity

%% Current States
v_x = p(1); %x velocity (m/s)
v_y = p(2); %y velocity (m/s)
phi = p(3); %phi (roll) (rad)
phi_d = p(4); %d(phi)/dt (roll rate) (rad/s)
psi = p(5); %psi (yaw) (rad)
psi_d = p(6); %d(psi)/dt (yaw rate) (rad/s)
a_x = acc_in(1); %x acceleration (m/s^2)
a_y = acc_in(2); %y accelerarion (m/s^2)
phi_dd = acc_in(4); %d^2(phi)/dt^2 (rad/s^2)
psi_dd = acc_in(5); %d^2(psi)/dt^2 (rad/s^2)

om = zeros([1,4]);

for i = 7:10

    om(i-6) = p(i); %angular speed of wheels (rad/s)

end
%% Car Physical Variables

l_fs = param.l_fs; %distance from front axle to sprung centre of mass (m)
l_rs = param.l_rs; %distance from rear axle to sprung centre of mass (m)
t_f = param.t_f; %front wheel track (m)
t_r = param.t_r; %rear wheel track (m)
h_f = param.h_f; %height of roll axis above ground at front axle (m)
h_r = param.h_r; %height of roll axis above ground at rear axle (m)
h_cgs = param.h_cgs; %height of sprung centre of mass above ground (m)
h_cguf = param.h_cguf; %height of front unsprung centre of mass above ground (m)
h_cgur = param.h_cgur; %height of rear unsprung centre of mass above ground (m)
M = param.M; %total mass (sprung + unsprung) (kg)
M_uf = param.M_uf; %front unsprung mass (kg) (I think of this is combined left and right)
M_ur = param.M_ur; %rear unsprung mass (kg)
I_xxs = param.I_xxs;    %
I_xys = param.I_xys;          %
I_xzs = param.I_xzs;    %sprung mass moment
I_yys = param.I_yys;   %of inertia tensor
I_yzs = param.I_yzs;          %
I_zzs = param.I_zzs;    %
I_zzuf = param.I_zzuf; %front unsprung mass moment of inertia
I_zzur = param.I_zzur; %rear unsprung mass moment of inertia
I_tlf = param.I_tlf; %
I_trf = param.I_trf; %moment of inertia of tyres
I_tlr = param.I_tlr; %(and I guess wheels too)
I_trr = param.I_trr; %

%spring/dampers
K_spf = param.K_spf; %front suspension stiffness (N/mm)
K_spr = param.K_spr; %rear suspension stiffness (N/mm)
B_f = param.B_f; %front suspension damping (Ns/mm)
B_r = param.B_r; %rear suspension damping (Ns/mm)

%anti-roll bars
K_rf = param.K_rf; %front anti-roll bar stiffness (Nm/rad)
K_rr = param.K_rr; %rear anti-roll bar stiffness (Nm/rad)

%roll stiffness
K_phif = param.K_phif; %(Nm/rad) not sure what 0.766 and 0.827 are
K_phir = param.K_phir; %(Nm/rad)
K_phi = param.K_phi;

%roll damping
B_phif = param.B_phif; %(Nms/rad) again, not sure about 0.766 and 0.827
B_phir = param.B_phir; %(Nms/rad)

K_sr = param.K_sr; %steering-to-wheel angle ratio (1/deg)

%tyre properties
t_wid = param.t_wid; %tyre width (m)
t_rad = param.t_rad; %tyre outer radius (m)
t_pressure = param.t_pressure; %tyre pressure (Pa)


%% Calculated Parameters
L = l_fs + l_rs; %wheelbase (m)
M_s = M - M_uf - M_ur; %sprung mass (kg) maybe should be factor of 2 in there???
l_cgs = (M_ur*l_rs - M_uf*l_fs)/M; %distance from total centre of mass to sprung centre of mass (m)
l_f = l_fs + l_cgs; %distance between front axle and total centre of mass (m)
l_r = l_rs - l_cgs; %distance between rear axle and total centre of mass (m)
M_f = M*l_r/L; %mass on front axle (kg)
M_r = M*l_f/L; %mass on reat axle (kg)
h_o = h_f + l_f*(h_r - h_f)/L; %height of roll axis above ground at total centre of mass (m)
h_s = h_cgs - h_o; %height of sprung centre of mass above roll axis (m)
h_uf = h_cguf - h_o; %height of front unsprung centre of mass above roll axis (m)
h_ur = h_cgur - h_o; %height of rear unsprung centre of mass above roll axis (m)
h_cg = (M_s*h_cgs + M_uf*h_cguf + M_ur*h_cgur)/M; %height of total centre of mass above ground (m)


%% Steering Inputs
d_steer = steer; %gets steering input

%% Calculate Internal Accelerations
%(V_0y = 0)
a_sx = a_x - psi_d*v_y - 2*h_s*phi_d*psi_d*cos(phi) - l_cgs*psi_d^2; %sprung mass x-acceleration (eqn 2.29)
a_sy = psi_d*v_x + l_cgs*psi_dd + h_s*cos(phi)*phi_dd - h_s*phi_d^2*sin(phi) - h_s*psi_d^2*sin(phi); %sprung mass y-acceleration (eqn 2.29)
a_ufx = a_x - l_f*psi_d^2; %front unsprung mass x-acceleration (eqn 2.16)
a_ufy = a_y + l_f*psi_dd; %front unsprung mass y-acceleration (eqn 2.16)
a_urx = a_x + l_r*psi_d^2; %rear unsprung mass x-acceleration (eqn 2.22)
a_ury = a_y - l_r*psi_dd; %rear unsprung mass y-acceleration (eqn 2.22)

%% Rotation Matrix
ROT = [1,0,0;...
    0,cos(phi),sin(phi);...
    0,-sin(phi),cos(phi)]; %eqn 2.39
I_b = [I_xxs+M_s*h_s^2,I_xys,I_xzs+M_s*h_s*l_cgs;...
    I_xys,I_yys+M_s*(h_s^2+l_cgs^2),I_yzs;...
    I_xzs+M_s*h_s*l_cgs,I_yzs,I_zzs+M_s*l_cgs^2]; %sprung mass inertia tensor (eqn 2.38)

I_c = ROT*I_b*ROT'; %chassis inertia tensor (eqn 2.40)
I_zzus = M_uf*l_f^2 + M_ur*l_r^2 + I_zzuf + I_zzur; %eqn 2.41
I_xxo = I_c(1,1);
I_zzo = I_c(3,3) + I_zzus; %effective I_zz (eqn 2.42)

%% Dynamic Weight Transfer Forces
Fzax = (M_s*h_s*a_sx + M_uf*h_uf*a_ufx + M_ur*h_ur*a_urx)/(2*L); %extra normal force from x-acceleration (eqn 2.50)
Fzayf = 1/t_f*(M_s*l_r*h_f/L*a_sy + M_uf*h_uf*a_ufy); %extra normal force on front axle from y-acceleration (eqn 2.51)
Fzayr = 1/t_r*(M_s*l_f*h_r/L*a_sy + M_ur*h_ur*a_ury); %extra normal force on rear axle from y-acceleration (eqn 2.52)
Fzphif = -1/t_f*(K_phif*phi + B_phif*phi_d); %extra normal force on front axle from roll (eqn 2.53)
Fzphir = -1/t_r*(K_phir*phi + B_phir*phi_d); %extra normal force on rear axle from roll (eqn 2.54)

%% Tyre Normal Forces
Fzlf = M*g*l_r/(2*L) - Fzax - Fzayf + Fzphif; %
Fzrf = M*g*l_r/(2*L) - Fzax + Fzayf - Fzphif; %total load on each tyre (eqns 2.55-58)
Fzlr = M*g*l_f/(2*L) + Fzax - Fzayr + Fzphir; %can probably add downforce term to these
Fzrr = M*g*l_f/(2*L) + Fzax + Fzayr - Fzphir; %

fz = [Fzlf, Fzrf, Fzlr, Fzrr];

%% Tyre Longitudinal/Lateral Forces
%left front wheel velocity  %
v_xlf = v_x + psi_d*t_f/2;  %
v_ylf = v_y + psi_d*l_f;    %
                            %
%right front wheel velocity %
v_xrf = v_x - psi_d*t_f/2;  %
v_yrf = v_y + psi_d*l_f;    %look at rotation (yaw) of car and draw triangles
                            %to see where these expressions come from
%left rear wheel velocity   %
v_xlr = v_x + psi_d*t_r/2;  %
v_ylr = v_y - psi_d*l_r;    %
                            %
%right rear wheel velocity  %
v_xrr = v_x - psi_d*t_r/2;  %
v_yrr = v_y - psi_d*l_r;    %

v_x = [v_xlf,v_xrf,v_xlr,v_xrr]; 

%tyre updates
% omega_lf = (v_xlf^2 + v_ylf^2)^(1/2); %
% omega_rf = (v_xrf^2 + v_yrf^2)^(1/2); %new wheel speeds
% omega_lr = (v_xlr^2 + v_ylr^2)^(1/2); %(omega is a misleading name)
% omega_rr = (v_xrr^2 + v_yrr^2)^(1/2); %

%get steering angle
delta = d_steer*pi/(180*K_sr); %gets steering angle from input (rad)
%beta = atan(v_y/v_x); %angle of vehicle velocity to direction of motion (rad)
beta_lf = atan(v_ylf/v_xlf); %angle of left front wheel to direction of motion (rad)
beta_rf = atan(v_yrf/v_xrf); %angle of right front wheel to direction of motion (rad)
beta_lr = atan(v_ylr/v_xlr); %angle of left rear wheel to direction of motion (rad)
beta_rr = atan(v_yrr/v_xrr); %angle of right rear wheel to direction of motion (rad)

%Slip Angles

a_lf = beta_lf - delta; %left front slip angle (rad)
a_rf = beta_rf - delta; %right front slip angle (rad)
a_lr = beta_lr; %left rear slip angle (rad)
a_rr = beta_rr; %right rear slip angle (rad)
slp_ang = [a_lf,a_rf,a_lr,a_rr]; %outputs slip angles

%%%  laplace_factor could be used to model response of tyre
%%%  currently not used


slp_rat = zeros([1 4]);
laplace_factor = zeros([1 4]);
rel_length = 0.25;

%%Slip Rates

for i = 1:4
    
    slp_rat(i) = (t_rad*om(i)-v_x(i))/abs(v_x(i));
    
    laplace_factor(i) = rel_length/(abs(om(i))*t_rad);
    
end


end

== matlab function AlexFullVehicleModel2018/Magic Formula for each Tyre/Subsystem/Lateral Magic Formula/MATLAB Function1 ==
  data: B input; LatForce output; C input; D input; E input; Mu input; Fz input; Slip input; fxt input; fxt0 input
function LatForce   = LatMagFormula(B,C,D,E,Mu,Fz,Slip,fxt,fxt0)

D_true = D*Mu*Fz;

LatForceTheory = -D_true*sin(C*atan(B*(1-E)*Slip+E*atan(B.*Slip)));
LatForce = LatForceTheory * (1 - (fxt/fxt0)^2)^(1/2);

== matlab function AlexFullVehicleModel2018/Magic Formula for each Tyre/Subsystem/Longitudinal Magic Formula/MATLAB Function1 ==
  data: B input; LongForce output; C input; D input; E input; Mu input; Fz input; Slip input; MaxLongForce output
function [LongForce,MaxLongForce]  = LongMagFormula(B,C,D,E,Mu,Fz,Slip)

D_true = D*Mu*Fz;

LongForce = D_true*sin(C*atan(B*(1-E)*Slip+E*atan(B.*Slip)));
MaxLongForce = D_true;
